simulink model "model_sinusoidal_gust_test"  (R2020b)
settings: configuration reference "Configuration" (kept outside this file)
settings Model: Creator=C:\Users\Dogukan  LastModifiedBy=dogukan
settings ConfigSetRef: SourceName=Configuration  SourceLocation=Base Workspace

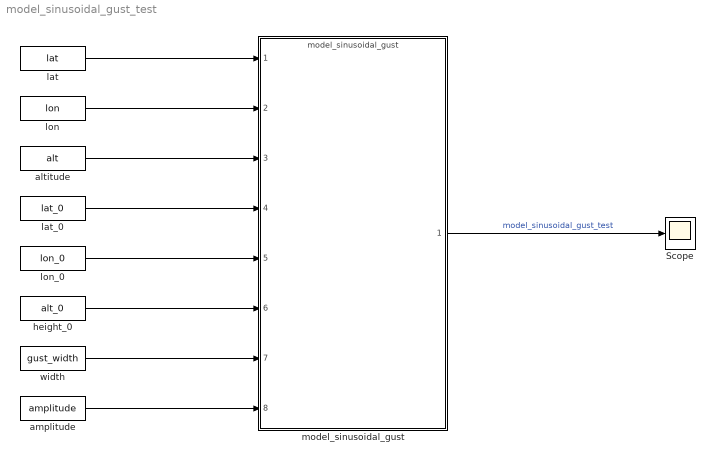
== system model_sinusoidal_gust_test ==
  Scope : Scope
  altitude : FromWorkspace  VariableName=alt
  amplitude : FromWorkspace  VariableName=amplitude
  height_0 : FromWorkspace  VariableName=alt_0
  lat : FromWorkspace  VariableName=lat
  lat_0 : FromWorkspace  VariableName=lat_0
  lon : FromWorkspace  VariableName=lon
  lon_0 : FromWorkspace  VariableName=lon_0
  model_sinusoidal_gust : ModelReference  ModelNameDialog=model_sinusoidal_gust.slx  SimulationMode=Normal  ModelReferenceVersion=1.73
  width : FromWorkspace  VariableName=gust_width
  wires:
  lat/1 -> model_sinusoidal_gust/1
  lon/1 -> model_sinusoidal_gust/2
  altitude/1 -> model_sinusoidal_gust/3
  model_sinusoidal_gust/1 -> Scope/1  "model_sinusoidal_gust_test"
  lat_0/1 -> model_sinusoidal_gust/4
  lon_0/1 -> model_sinusoidal_gust/5
  height_0/1 -> model_sinusoidal_gust/6
  width/1 -> model_sinusoidal_gust/7
  amplitude/1 -> model_sinusoidal_gust/8
